simulink model "Global_Control"  (R2016a)
settings: Solver=ode8  StartTime=0.0  StopTime=1400  FixedStep=1  RelTol=1e-3
(part 2 of 2)

== matlab function Global_Control/Controller1 ==
  data: Wetland_Height input; Q1 output; C1 input; C2 input; H1 input; H2 input; Q3 input; Q2 output
function [Q1,Q2] = Controller(Wetland_Height,C1,C2,H1,H2,Q3)

Volume=Wetland_Height*1000; % Observe water level in wetland to extimate height

if Q3 > 0
    if Volume < 2000 
        Volume_Difference= 2000 - Volume;
        Temp1=Volume_Difference-Q3;
        if Temp1 > 0;
            Q1=C1/(C1+C2)*Temp1; % Split the flows based on Conctration ratio
            Q2=C2/(C1+C2)*Temp1;
        else
            Q1=0;
            Q2=0;
        end  
    else
        Q1=0;
        Q2=0;
    end
else   % Maintain a level in ponds 
    if H1 > 1.5 && H2>0.80
        Q1=3*C1/(C1+C2);
        Q2=3*C2/(C1+C2);
    elseif H1 > 1.5 
        Q1=3;
        Q2=0;
    elseif H2 > 1
        Q2=3;
        Q1=0;
    else
        Q1=0;
        Q2=0;
    end

end

== matlab function Global_Control/Subsystem2/ Ammonia - Nitrate - Interface ==
  data: C_am input; C_nit output; Cni input; Cam input
function C_nit = fcn(C_am,Cni,Cam)
C_nit=abs(C_am- Cam)+Cni;

== matlab function Global_Control/Subsystem2/ Ammonia and Nitrate  ==
  data: C1 input; C2 input; C3 input; v input; dc1 output; Cint input; Qi input; Qout input; dv input; k_am input; dc2 output; k_ni input; k_TSS input; dc3 output
function [dc1,dc2,dc3] = Nitrogen_Cycle(C1,C2,C3,v,Cint,Qi,Qout,dv,k_am,k_ni,k_TSS)

A=[Qi   0  0;
    0   Qi 0;
    0   0  Qi];

B=[Qout + dv + k_am*v    0               0;
    0              Qout + dv + k_ni*v    0;
    0                  0               Qout + dv + k_TSS*v ];

C=[C1;
   C2;
   C3];

if v==0
    dc1=0;
    dc2=0;
    dc3=0;
else 
    dc=(A*Cint - B*C)*(1/v);
    dc1=dc(1);
    dc2=dc(2);
    dc3=dc(3);

end

== matlab function Global_Control/Subsystem2/ Concentration  ==
  data: Nitrate input; Ammonia input; TSS input; C output; Qin input
function C = fcn(Nitrate,Ammonia,TSS,Qin)

if Qin>0
    C=[Ammonia; Nitrate;TSS];
else
    C=[0; 0; 0];
    
end

== matlab function Global_Control/Subsystem2/Height and Volume ==
  data: Qin input; A input; dH output; Qout input
function dH  = Height_and_Volume(Qin,A,Qout)
    dH = (Qin-Qout)*(1/A);
end

== matlab function Global_Control/Subsystem2/Overflow  ==
  data: H input; Q_overflow output; Qin input; Overflow_Height input
function Q_overflow = fcn(H,Qin,Overflow_Height)
%#codegen
if H>=Overflow_Height;
    Q_overflow=Qin;
else 
    Q_overflow=0;
end

== matlab function Global_Control/Subsystem2/Oxygen Control/ Oxygen Setpoint1 ==
  data: Height input; Intergration_Control output; Integration_Control1 output; Integration_Control2 output
function [Intergration_Control,Integration_Control1,Integration_Control2] = fcn(Height)
if Height>0 
    Intergration_Control=0;
else 
    Intergration_Control=1;
end
    
if Height>0.25
    Integration_Control1=0;
else 
    Integration_Control1=1;
end
if Height>0.75
    Integration_Control2=0;
else 
    Integration_Control2=1;
end

== matlab function Global_Control/Subsystem2/Oxygen Control/0 to 0.25/ Nitrate ==
  data: Oxygen_Level input; K_Nitrate output; K_Nitr input
function K_Nitrate = fcn(Oxygen_Level,K_Nitr)

if Oxygen_Level< 1.0
    K_Nitrate = K_Nitr;
else
    K_Nitrate = 0;
end

== matlab function Global_Control/Subsystem2/Oxygen Control/0 to 0.25/ Oxygen Control ==
  data: c input; dOxygen_Level output; K input
function dOxygen_Level = fcn(c,K)

dOxygen_Level = -c * K;

== matlab function Global_Control/Subsystem2/Q out ==
  data: H input; Qout output; Control_Height input
function Qout = fcn(H,Control_Height)

if H<=Control_Height
    Qout=0;
else
   
        Qout = sqrt(2*9.81*H);
   

end

== matlab function Global_Control/Subsystem1/Oxygen Control/0.25 ro 0.75/ Nitrate ==
  data: Oxygen_Level input; K_Nitrate output; K_Nitr input
function K_Nitrate = fcn(Oxygen_Level,K_Nitr)

if Oxygen_Level< 1.0
    K_Nitrate = K_Nitr;
else
    K_Nitrate = 0;
end

== matlab function Global_Control/Subsystem1/Oxygen Control/0.25 ro 0.75/ Oxygen Control ==
  data: c input; dOxygen_Level output; K input
function dOxygen_Level = fcn(c,K)

dOxygen_Level = -c * K;

== matlab function Global_Control/Subsystem1/Oxygen Control/0.75 / Nitrate ==
  data: Oxygen_Level input; K_Nitrate output; K_Nitr input
function K_Nitrate = fcn(Oxygen_Level,K_Nitr)

if Oxygen_Level< 1.0
    K_Nitrate = K_Nitr;
else
    K_Nitrate = 0;
end

== matlab function Global_Control/Subsystem1/Oxygen Control/0.75 / Oxygen Control ==
  data: c input; dOxygen_Level output; K input
function dOxygen_Level = fcn(c,K)

dOxygen_Level = -c * K;

== matlab function Global_Control/Subsystem3/Oxygen Control/0.25 ro 0.75/ Nitrate ==
  data: Oxygen_Level input; K_Nitrate output; K_Nitr input
function K_Nitrate = fcn(Oxygen_Level,K_Nitr)

if Oxygen_Level< 1.0
    K_Nitrate = K_Nitr;
else
    K_Nitrate = 0;
end

== matlab function Global_Control/Subsystem3/Oxygen Control/0.25 ro 0.75/ Oxygen Control ==
  data: c input; dOxygen_Level output; K input
function dOxygen_Level = fcn(c,K)

dOxygen_Level = -c * K;

== matlab function Global_Control/Subsystem3/Oxygen Control/0.75 / Nitrate ==
  data: Oxygen_Level input; K_Nitrate output; K_Nitr input
function K_Nitrate = fcn(Oxygen_Level,K_Nitr)

if Oxygen_Level< 1.0
    K_Nitrate = K_Nitr;
else
    K_Nitrate = 0;
end

== matlab function Global_Control/Subsystem3/Oxygen Control/0.75 / Oxygen Control ==
  data: c input; dOxygen_Level output; K input
function dOxygen_Level = fcn(c,K)

dOxygen_Level = -c * K;

== matlab function Global_Control/Subsystem2/Oxygen Control/0.25 ro 0.75/ Nitrate ==
  data: Oxygen_Level input; K_Nitrate output; K_Nitr input
function K_Nitrate = fcn(Oxygen_Level,K_Nitr)

if Oxygen_Level< 1.0
    K_Nitrate = K_Nitr;
else
    K_Nitrate = 0;
end

== matlab function Global_Control/Subsystem2/Oxygen Control/0.25 ro 0.75/ Oxygen Control ==
  data: c input; dOxygen_Level output; K input
function dOxygen_Level = fcn(c,K)

dOxygen_Level = -c * K;

== matlab function Global_Control/Subsystem2/Oxygen Control/0.75 / Nitrate ==
  data: Oxygen_Level input; K_Nitrate output; K_Nitr input
function K_Nitrate = fcn(Oxygen_Level,K_Nitr)

if Oxygen_Level< 1.0
    K_Nitrate = K_Nitr;
else
    K_Nitrate = 0;
end

== matlab function Global_Control/Subsystem2/Oxygen Control/0.75 / Oxygen Control ==
  data: c input; dOxygen_Level output; K input
function dOxygen_Level = fcn(c,K)

dOxygen_Level = -c * K;

== matlab function Global_Control/Wetland/Oxygen Control/0.25 ro 0.75/ Nitrate ==
  data: Oxygen_Level input; K_Nitrate output; K_Nitr input
function K_Nitrate = fcn(Oxygen_Level,K_Nitr)

if Oxygen_Level< 1.0
    K_Nitrate = K_Nitr;
else
    K_Nitrate = 0;
end

== matlab function Global_Control/Wetland/Oxygen Control/0.25 ro 0.75/ Oxygen Control ==
  data: c input; dOxygen_Level output; K input
function dOxygen_Level = fcn(c,K)

dOxygen_Level = -c * K;

== matlab function Global_Control/Wetland/Oxygen Control/0.75 / Nitrate ==
  data: Oxygen_Level input; K_Nitrate output; K_Nitr input
function K_Nitrate = fcn(Oxygen_Level,K_Nitr)

if Oxygen_Level< 1.0
    K_Nitrate = K_Nitr;
else
    K_Nitrate = 0;
end

== matlab function Global_Control/Wetland/Oxygen Control/0.75 / Oxygen Control ==
  data: c input; dOxygen_Level output; K input
function dOxygen_Level = fcn(c,K)

dOxygen_Level = -c * K;

== matlab function Global_Control/Wetland/Oxygen Control/0.75 1/ Nitrate ==
  data: Oxygen_Level input; K_Nitrate output; K_Nitr input
function K_Nitrate = fcn(Oxygen_Level,K_Nitr)

if Oxygen_Level< 1.0
    K_Nitrate = K_Nitr;
else
    K_Nitrate = 0;
end

== matlab function Global_Control/Wetland/Oxygen Control/0.75 1/ Oxygen Control ==
  data: c input; dOxygen_Level output; K input
function dOxygen_Level = fcn(c,K)

dOxygen_Level = -c * K;

== matlab function Global_Control/Subsystem1/Zero Check ==
  data: c input; cout output; v input
function cout = zero(c,v)

if v > 0
    cout = c;
else
    cout = 0;
end

== matlab function Global_Control/Subsystem3/Zero Check1 ==
  data: c input; cout output; v input
function cout = zero(c,v)

if v > 0
    cout = c;
else
    cout = 0;
end

== matlab function Global_Control/Subsystem2/Zero Check1 ==
  data: c input; cout output; v input
function cout = zero(c,v)

if v > 0
    cout = c;
else
    cout = 0;
end

== matlab function Global_Control/Wetland/Zero Check ==
  data: c input; cout output; v input
function cout = zero(c,v)

if v > 0
    cout = c;
else
    cout = 0;
end
